simulink model "ABS"  (R2018a)
settings: Solver=ode23s  StartTime=0.0  StopTime=50  MaxStep=0.5  RelTol=1e-6
values from neighbouring files (symbols this model uses):
  Brake_torque_max = 1300    [ABS_parameters.m]
  g = 9.81    [ABS_parameters.m]
  J = 0.288    [ABS_parameters.m]
  m = 1310    [ABS_parameters.m]
  mu = [0 0.4 0.8 0.97 1 1 0.96 0.94 0.92 0.9 0.88 0.855 ... (21 elements, 1x21)]    [mu.mat]
  R = 0.3    [ABS_parameters.m]
  slip = [0 0.05 0.1 0.15 0.2 0.25 0.3 0.35 0.4 0.45 0.5 0.55 ... (21 elements, 1x21)]    [slip.mat]
  V = 44    [ABS_parameters.m]
libraries: simulink x1
settings Model: Creator=Saurabh Suman  LastModifiedBy=Saurabh Suman

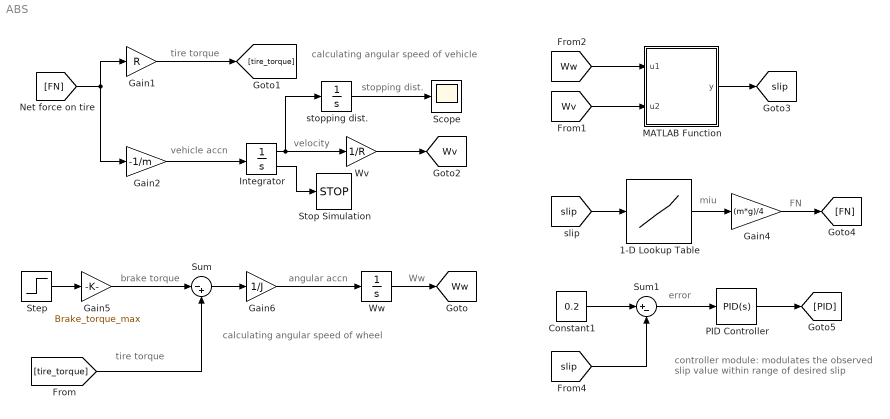
== system ABS ==
  note: stopping dist.
  note: controller module: modulates the observed
      |  slip value within range of desired slip
  note: error
  note: FN
  note: miu
  note: calculating angular speed of wheel
  note: calculating angular speed of vehicle
  note: velocity
  note: vehicle accn
  note: Ww
  note: angular accn
  note: tire torque
  note: brake torque
  note: tire torque
  1-D Lookup Table : Lookup_n-D  NumberOfTableDimensions=1  BreakpointsForDimension1=slip  Table=mu  InternalRulePriority=Speed  RndMeth=Simplest  InputSameDT=on
  Constant1 : Constant  Value=0.2
  Gain1 : Gain  Gain=R
  Gain2 : Gain  Gain=-1/m
  Gain4 : Gain  Gain=(m*g)/4
  Gain5 : Gain  Gain=Brake_torque_max
  Gain6 : Gain  Gain=1/J
  Integrator : Integrator  InitialCondition=V  LimitOutput=on  LowerSaturationLimit=0  ShowSaturationPort=on
  MATLAB Function : MATLAB Function  TreatAsAtomicUnit=on
  PID Controller : simulink/Continuous/PID Controller  Controller=PID  TimeDomain=Continuous-time  SampleTime=-1  IntegratorMethod=Forward Euler  FilterMethod=Forward Euler  Form=Parallel  UseFilter=on  ControllerParametersSource=internal  P=1  I=1  D=0  N=100  InitialConditionSource=internal  InitialConditionForIntegrator=0  InitialConditionForFilter=0  ExternalReset=none  LimitOutput=off  UpperSaturationLimit=inf  LowerSaturationLimit=-inf  LinearizeAsGain=on  AntiWindupMode=none  Kb=1  TrackingMode=off  Kt=1  PParamMin=[]  PParamMax=[]  IParamMin=[]  IParamMax=[]  DParamMin=[]  DParamMax=[]  NParamMin=[]  NParamMax=[]  KbParamMin=[]  KbParamMax=[]  KtParamMin=[]  KtParamMax=[]  POutMin=[]  POutMax=[]  IOutMin=[]  IOutMax=[]  DOutMin=[]  DOutMax=[]  NOutMin=[]  NOutMax=[]  KbOutMin=[]  KbOutMax=[]  KtOutMin=[]  KtOutMax=[]  IntegratorOutMin=[]  IntegratorOutMax=[]  FilterOutMin=[]  FilterOutMax=[]  SumOutMin=[]  SumOutMax=[]  SumI1OutMin=[]  SumI1OutMax=[]  SumI2OutMin=[]  SumI2OutMax=[]  SumI3OutMin=[]  SumI3OutMax=[]  SumDOutMin=[]  SumDOutMax=[]  SaturationOutMin=[]  SaturationOutMax=[]  IntegratorContinuousStateAttributes=''  IntegratorStateMustResolveToSignalObject=off  IntegratorRTWStateStorageClass=Auto  FilterContinuousStateAttributes=''  FilterStateMustResolveToSignalObject=off  FilterRTWStateStorageClass=Auto  DifferentiatorICPrevScaledInput=0  DifferentiatorOutMin=[]  DifferentiatorOutMax=[]  FilterDiffOutCoefMin=[]  FilterDiffOutCoefMax=[]  SumDenOutMin=[]  SumDenOutMax=[]  SumNumOutMin=[]  SumNumOutMax=[]  ReciprocalOutMin=[]  ReciprocalOutMax=[]  DivideOutMin=[]  DivideOutMax=[]  TunerSelectOption=Transfer Function Based (PID Tuner App)
  Scope : Scope
  Step : Step  Time=0  SampleTime=0
  Stop Simulation : Stop
  Sum : Sum  Inputs=|-+
  Sum1 : Sum  Inputs=|+-
  Wv : Gain  Gain=1/R
  Ww : Integrator  LimitOutput=on  UpperSaturationLimit=V/R  LowerSaturationLimit=0
  stopping dist. : Integrator
  tag scope: Wv=global, Ww=global, slip=global
  wires:
  Gain5/1 -> Sum/1
  [tire_torque] -> Sum/2
  Sum/1 -> Gain6/1
  Gain6/1 -> Ww/1
  Ww/1 -> [Ww]
  [FN] -> Gain2/1, Gain1/1
  Gain1/1 -> [tire_torque]
  Gain2/1 -> Integrator/1
  Integrator/1 -> stopping dist./1, Wv/1
  Wv/1 -> [Wv]
  Integrator/2 -> Stop Simulation/1
  [Ww] -> MATLAB Function/1(u1)
  [Wv] -> MATLAB Function/2(u2)
  MATLAB Function/1(y) -> [slip]
  [slip] -> 1-D Lookup Table/1
  1-D Lookup Table/1 -> Gain4/1
  Gain4/1 -> [FN]
  Constant1/1 -> Sum1/1
  [slip] -> Sum1/2
  Sum1/1 -> PID Controller/1
  PID Controller/1 -> [PID]
  Step/1 -> Gain5/1
  stopping dist./1 -> Scope/1

== matlab function ABS/MATLAB Function ==
  data: u1 input; y output; u2 input
function y = fcn(u1, u2)
if u1>u2
    y=(1.0 - u2/(u1 + (u1==0)*eps));
else
    y=(1.0 - u1/(u2 + (u2==0)*eps));
end
